simulink model "Computer_Exercise_EKF_Implementation_v2019b"  (R2025b)
settings: Solver=ode15s  StartTime=0.0  StopTime=20.0  RelTol=1e-6  EnableMultiTasking=on
settings Model: Creator=mangold  LastModifiedBy=navya
settings SolverCC: AlgebraicLoopSolver=TrustRegion
settings DataIOCC: LimitDataPoints=on  SaveFormat=Array  SignalLoggingSaveFormat=ModelDataLogs  ReturnWorkspaceOutputs=off
settings OptimizationCC: ExpressionDepthLimit=2147483647.0  LifeSpan=inf
settings DebuggingCC: UnderspecifiedInitializationDetection=Classic  MergeDetectMultiDrivingBlocksExec=none  SolverPrmCheckMsg=warning  FcnCallInpInsideContextMsg=warning  UnconnectedInputMsg=warning  UnconnectedOutputMsg=warning  UnconnectedLineMsg=warning  StateNameClashWarn=warning  SFUnexpectedBacktrackingDiag=warning  SFNoUnconditionalDefaultTransitionDiag=warning  SFExecutionAtInitializationDiag=none  ArithmeticOperatorsInVariantConditions=warning
settings HardwareCC: ProdBitPerPointer=32.0  ProdBitPerSizeT=32.0  ProdBitPerPtrDiffT=32.0  ProdLargestAtomicFloat=None  ProdIntDivRoundTo=Undefined  ProdEndianess=Unspecified  ProdWordSize=32.0  ProdHWDeviceType=32-bit Generic
settings ModelReferenceCC: EnableRefExpFcnMdlSchedulingChecks=on  PropagateSignalLabelsOutOfModel=off
settings SFSimCC: SimUseLocalCustomCode=off  CustomCodeUndefinedFunction=UseInterfaceOnly
settings RTWCC: RTWUseLocalCustomCode=off  GPUComputeCapability=3.5
settings CodeAppCC: StateflowObjectComments=on
settings GRTTargetCC: TargetLangStandard=C89/C90 (ANSI)  CombineOutputUpdateFcns=off  GRTInterface=on
settings ConfigComp: CovMetricSettings=dw  CovSaveCumulativeToWorkspaceVar=on  CovSaveSingleToWorkspaceVar=on  CovExternalEMLEnable=off

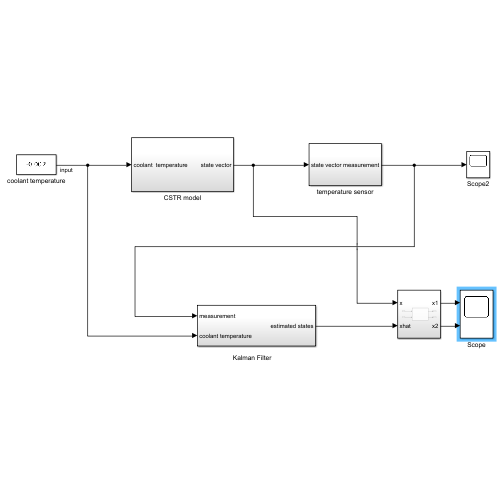
[thumbnail: Simulink's stored preview of the top-level diagram]
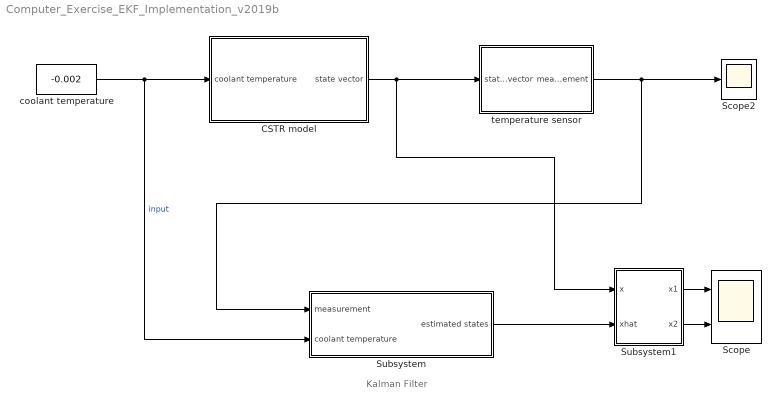
== system Computer_Exercise_EKF_Implementation_v2019b ==
  note: Kalman Filter
  CSTR model : Subsystem
  Scope : Scope  NumInputPorts=2
      settings: ActiveDisplayYMinimum=-0.12389  ActiveDisplayYMaximum=1.11503
  Scope2 : Scope
      settings: ActiveDisplayYMinimum=-7.83685  ActiveDisplayYMaximum=10.35542  DataLoggingVariableName=ScopeData2
  Subsystem : Subsystem
  Subsystem1 : Subsystem
  coolant temperature : Constant  Value=-0.002
  temperature sensor : Subsystem
  wires:
  coolant temperature/1 -> CSTR model/1(coolant temperature), Subsystem/2(coolant temperature)  "input"
  CSTR model/1(state vector) -> Subsystem1/1(x), temperature sensor/1(state vector)
  temperature sensor/1(measurement) -> Scope2/1, Subsystem/1(measurement)
  Subsystem1/2(x2) -> Scope/2
  Subsystem1/1(x1) -> Scope/1
  Subsystem/1(estimated states) -> Subsystem1/2(xhat)

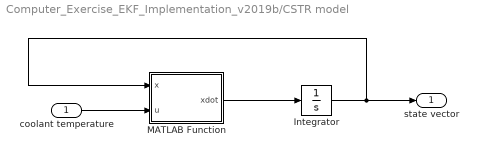
== system Computer_Exercise_EKF_Implementation_v2019b/CSTR model ==
  coolant temperature : Inport
  Integrator : Integrator  InitialCondition=[0.5, 0]
  MATLAB Function : MATLAB Function  TreatAsAtomicUnit=on
  state vector : Outport
  wires:
  MATLAB Function/1(xdot) -> Integrator/1
  coolant temperature/1 -> MATLAB Function/2(u)
  Integrator/1 -> MATLAB Function/1(x), state vector/1

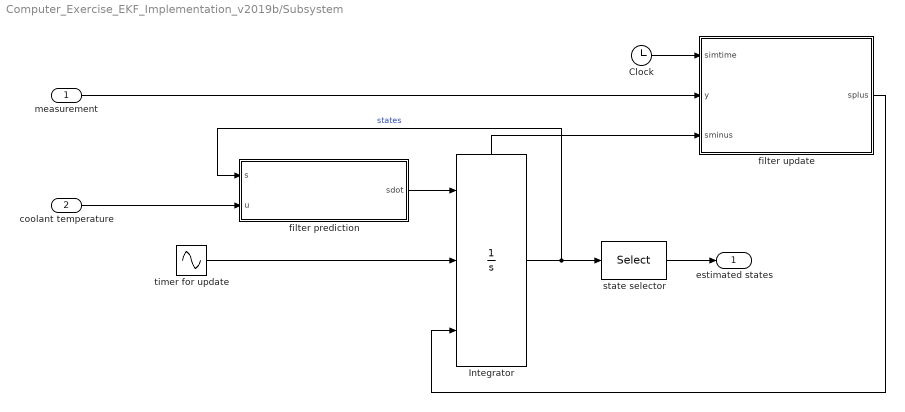
== system Computer_Exercise_EKF_Implementation_v2019b/Subsystem ==
  measurement : Inport
  coolant temperature : Inport  Port=2
  Clock : Clock
  Integrator : Integrator  ExternalReset=rising  InitialConditionSource=external  InitialCondition=[0.5; 0; 1; 0; 0; 1]  ShowStatePort=on
  filter prediction : MATLAB Function  TreatAsAtomicUnit=on
  filter update : MATLAB Function  TreatAsAtomicUnit=on
  state selector : Selector  InputPortWidth=6  IndexOptions=Index vector (dialog)  Indices=[1 2]  OutputSizes=1
  timer for update : Sin  Frequency=2*pi/0.1  Phase=-1.0e-04  SampleTime=0
  estimated states : Outport
  wires:
  filter prediction/1(sdot) -> Integrator/1
  Integrator/1 -> filter prediction/1(s), state selector/1  "states"
  filter update/1(splus) -> Integrator/3
  timer for update/1 -> Integrator/2
  coolant temperature/1 -> filter prediction/2(u)
  measurement/1 -> filter update/2(y)
  Integrator/State -> filter update/3(sminus)
  state selector/1 -> estimated states/1
  Clock/1 -> filter update/1(simtime)

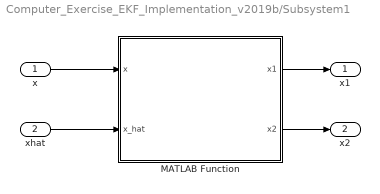
== system Computer_Exercise_EKF_Implementation_v2019b/Subsystem1 ==
  x : Inport
  xhat : Inport  Port=2
  MATLAB Function : MATLAB Function  TreatAsAtomicUnit=on
  x1 : Outport
  x2 : Outport  Port=2
  wires:
  x/1 -> MATLAB Function/1(x)
  xhat/1 -> MATLAB Function/2(x_hat)
  MATLAB Function/1(x1) -> x1/1
  MATLAB Function/2(x2) -> x2/1

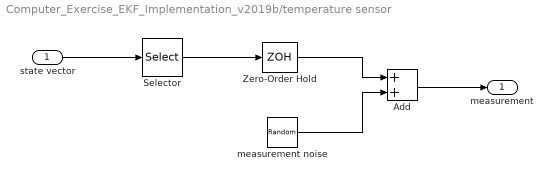
== system Computer_Exercise_EKF_Implementation_v2019b/temperature sensor ==
  state vector : Inport
  Add : Sum
  Selector : Selector  InputPortWidth=2  IndexOptions=Index vector (dialog)  Indices=[2]  OutputSizes=1
  Zero-Order Hold : ZeroOrderHold  SampleTime=0.1
  measurement noise : RandomNumber  Variance=1e-4  SampleTime=0.1
  measurement : Outport
  wires:
  Selector/1 -> Zero-Order Hold/1
  Zero-Order Hold/1 -> Add/1
  measurement noise/1 -> Add/2
  state vector/1 -> Selector/1
  Add/1 -> measurement/1

== matlab function Computer_Exercise_EKF_Implementation_v2019b/Subsystem/filter prediction ==
  data: s input; u input; sdot output
function sdot = CSTR_EKF_predictor(s,u)
%
% right-hand sides of ODEs for EKF prediction step

    %% rename state variables
    x1 = s(1);
    x2 = s(2);
    P  = reshape(s(3:6),2,2);
    
    %% process noise spectral density matrix
    Q = zeros(2,2);
    
    %% define model parameters
    a1 = 0.2674;
    a2 = 1.815;
    b1 = 1.05e+14;
    b2 = 4.92e+13;
    g  = 1.5476;
    E  = 34.2583;
    
    %% compute reaction rate
    r = (1-x1) * exp(-E/(1+x2));

    %% compute right-hand sides of balance equations
    x1dot = -a1*x1 + b1*r;
    x2dot = -a2*x2 + b2*r + g*u;
    
    %% compute jacobian of the system
    J=zeros(2,2);

    J(1,1) = -a1 - b1/exp(E/(1 + x2));
    J(1,2) = (b1*E*(1 - x1))/(exp(E/(1 + x2))*(1 + x2)^2);
    J(2,1) = -(b2/exp(E/(1 + x2)));
    J(2,2) = -a2 + (b2*E*(1 - x1))/...
              (exp(E/(1 + x2))*(1 + x2)^2);
    
    %% compute time derivatives of estimation error
    Pdot = J*P + P *J' + Q;
    
sdot = [x1dot; x2dot; reshape(Pdot,4,1)];

== matlab function Computer_Exercise_EKF_Implementation_v2019b/CSTR model/MATLAB Function ==
  data: x input; u input; xdot output
function xdot = CSTR_rhs(x,u)
%
%  right-hand sides of CSTR model equations

%% define model parameters
    a1 = 0.2674;
    a2 = 1.815;
    b1 = 1.05e+14;
    b2 = 4.92e+13;
    g  = 1.5476;
    E  = 34.2583;
    
%% compute reaction rate
    r = (1-x(1)) * exp(-E/(1+x(2)));

%% compute right-hand sides of balance equations
    x1dot = -a1*x(1) + b1*r;
    x2dot = -a2*x(2) + b2*r + g*u;

xdot = [x1dot; x2dot];

== matlab function Computer_Exercise_EKF_Implementation_v2019b/Subsystem/filter update ==
  data: simtime input; y input; sminus input; splus output
function splus = CSTR_EKF_update(simtime,y,sminus)
%
% update step of Extended Kalman Filter

  if simtime>1e-3
    %% rename state variables
    xminus = sminus(1:2);
    Pminus = reshape(sminus(3:6),2,2);
    
    %% variance of measurement noise
    R = 1e-4;
    
    %% compute simulated measurement signal
    dh_dx = [0 1];
    yhat = dh_dx*xminus;
    
    %% compute filter gain
    Pxy   = Pminus*dh_dx';
    Pyy   = dh_dx*Pminus*dh_dx' + R;
    Kgain = Pxy/Pyy;
    
    %% update states and estimation error matrix
    xplus = xminus + Kgain*( y - yhat );
    Pplus = Pminus - Kgain*Pyy*Kgain';
    
  else
    %% initial guess of x and P
    xplus=[0; 0];
    Pplus=diag([0.25,0.25]);
  end

splus = [xplus;reshape(Pplus,4,1)];

== matlab function Computer_Exercise_EKF_Implementation_v2019b/Subsystem1/MATLAB Function ==
  data: x input; x1 output; x_hat input; x2 output
function [x1,x2] = sys_state_comparison(x,x_hat)


x1 = [x(1), x_hat(1)];
x2 = [x(2), x_hat(2)];
